simulink library "vec"  (Simulink 8.1)
settings: Solver=ode1  StartTime=0.0  StopTime=Inf  FixedStep=0.001  RelTol=1e-3
PostLoadFcn:
  | , if any(exist('dsrtsu_mdlpostloadfcn', 'file') == [2, 3, 6]), try dsrtsu_mdlpostloadfcn('Execute', bdroot); catch fprintf('Error in PostLoadFcn (dsrtsu_mdlpostloadfcn) for model "%s":\n %s\n', bdroot, lasterr); end, end,
libraries: hcu_lib x2
settings Model: DSRTSU_INTERNAL_RTI_VER=450  DSRTSU_INTERNAL_RTI_TYPE=rti1401  RTICANMMDATA=struct('GeneralSetupData',struct('modelroot','D:\PROJECTS\HAITEC\TAIWAN_HAITEC_SVN\trunk\AdasDragon\software\sw_development\arch\app\ifo','generalsettings',struct('filesettings',struct('destfolder',struct('Name','RTICANMM_FILES','Check',1),'buildfolder',struct('Name','.','Check',1),'AbsDestfolder',struct('Name','D:\PROJECTS\HAITEC\TAIWAN_HAITEC_SVN\trunk\AdasDragon\software\sw_development\arch\app\ifo\RTICANMM_FILES'),'AbsBuildfolder',struct('Name','D:\PROJECTS\HAITEC\TAIWAN_HAITEC_SVN\trunk\AdasDragon\software\sw_development\arch\app\ifo'))),'options',struct('addpaths',1,'rmpaths',1,'addtrcexclusion',logical(1),'cannavigator',struct('checkmonitoring',0),'show_usrtrc',0,'use_usrtrc',0),'advanced',struct('options',[1 1 1 1 1 1 1 1 1 1 1 1 1 1 1 1 1 1 1 1 1 1 1 1 1 1 1 1 1 1 1 1 1 1 1 1 1 1 1 1 1 1 1 1 1 1 1 1 1 1 1 1 1 1 1 1 1 1 1 1 1 1 1 1 1 1 1 1 1 1 1 1 1 1 1 1 1 1 1 1 1 1 1 1 1 1 1 1 1 1 1 1 1 1 1 1 1 1 1 1]),'MPSetup',{{}},'modelname','vec','block','vec'))  DSRTSU_INTERNAL_RTIFPGA=40  Creator=AT015411  LastModifiedBy=tescamilla

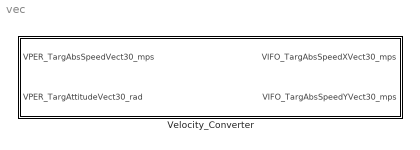
== system vec ==
  Velocity_Converter : Subsystem

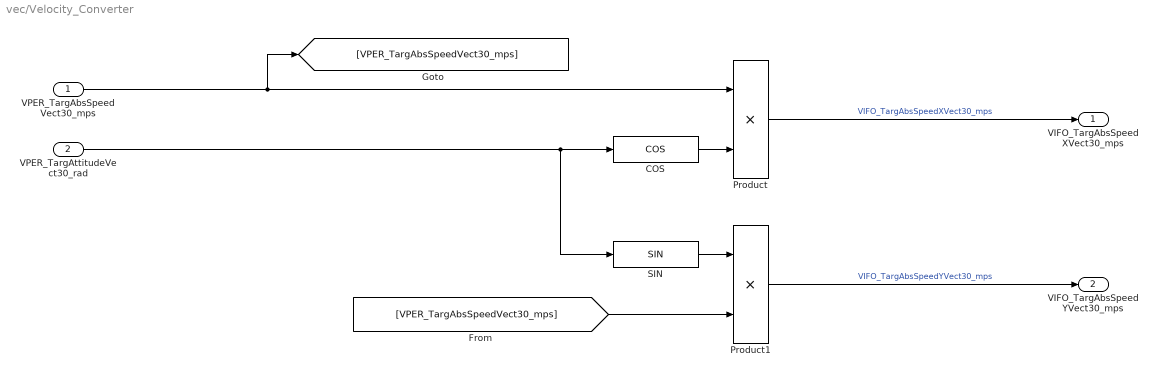
== system vec/Velocity_Converter ==
  VPER_TargAbsSpeedVect30_mps : Inport
  VPER_TargAttitudeVect30_rad : Inport  Port=2
  COS : hcu_lib/COS
  Product : Product
  Product1 : Product
  SIN : hcu_lib/SIN
  VIFO_TargAbsSpeedXVect30_mps : Outport
  VIFO_TargAbsSpeedYVect30_mps : Outport  Port=2
  wires:
  Product1/1 -> VIFO_TargAbsSpeedYVect30_mps/1  "VIFO_TargAbsSpeedYVect30_mps"
  [VPER_TargAbsSpeedVect30_mps] -> Product1/2
  SIN/1 -> Product1/1
  COS/1 -> Product/2
  VPER_TargAttitudeVect30_rad/1 -> COS/1, SIN/1
  VPER_TargAbsSpeedVect30_mps/1 -> Product/1, [VPER_TargAbsSpeedVect30_mps]
  Product/1 -> VIFO_TargAbsSpeedXVect30_mps/1  "VIFO_TargAbsSpeedXVect30_mps"
